simulink library "Susp_LUT"  (R2023b)
settings: Solver=VariableStepAuto  StartTime=0.0  StopTime=10.0  RelTol=1e-3
undefined symbols (not defined in the file or in its folder): Axle1D, AxleIn, Init, RaceFix, RaceSpin, Susp, Visual, X, Y, Z
libraries: Susp_DOF15 x5, LUT_Susp_Lib x2, sm_lib x2, Suspension_Utilities x2, Steer_Ackermann x1, Steer_Control_Axle2 x1
Description:
  | Component of Simscape Vehicle Templates Library
  | 
  | Copyright 2018-2026 The MathWorks, Inc.
settings Model: Creator=smiller  LastModifiedBy=smiller
settings ModelReferenceCC: EnableRefExpFcnMdlSchedulingChecks=on

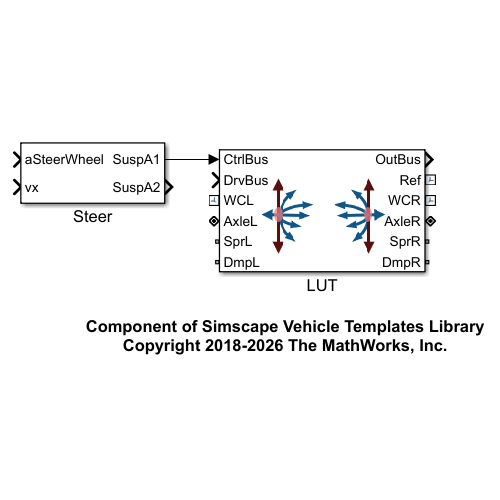
[thumbnail: Simulink's stored preview of the top-level diagram]
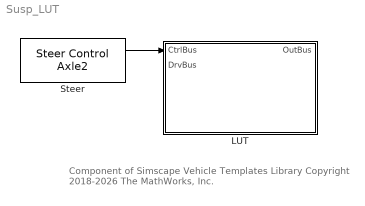
== system Susp_LUT ==
  note: Component of Simscape Vehicle Templates Library
      | Copyright 2018-2026 The MathWorks, Inc.
  LUT : Subsystem  mask(LUT Suspension with Optional Compliance and Steering){}
      mask help: Models suspension kinematics defined using a lookup table. The wheel frame lateral position, longitudinal position, and orientation are defined based on the height of the wheel frame. An optional 6-DOF compliance is placed at the wheel frame. Steering can be enabled.
      mask Display: image('sm_car_vehicle_susp_lut_IMAGE.png');
  Steer : Steer_Control_Axle2/Steer Control Axle2  Steer=Control.Default.Steer
  wires:
  Steer/1 -> LUT/1(CtrlBus)

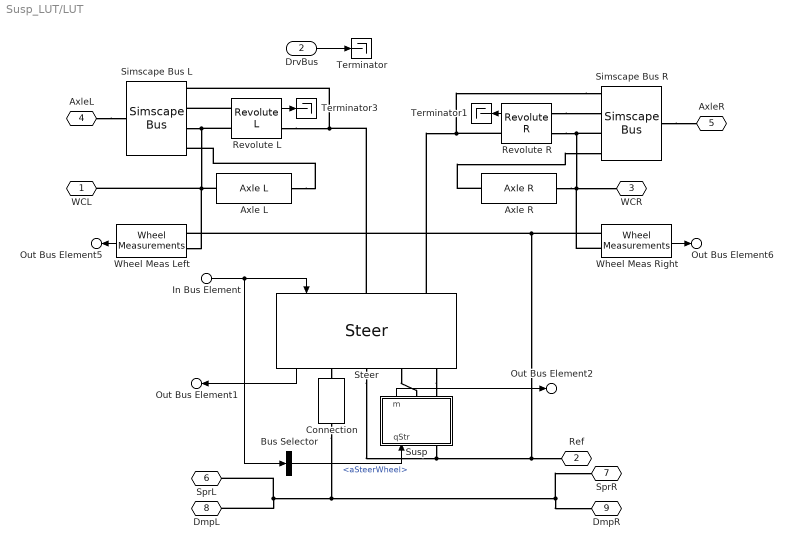
== system Susp_LUT/LUT ==
  In Bus Element : Inport  PortName=CtrlBus  Element=Steer
  DrvBus : Inport  Port=2
  Axle L : Susp_DOF15/Simple/Axle L  axle_len=Susp.LUT.Axle.xAxle.Value  axle_mass=Susp.LUT.Axle.mAxle.Value  clr_axle=Visual.Axle.clr  opc_axle=Visual.part.opc  radius_axle=Visual.Axle.rad
  Axle R : Susp_DOF15/Simple/Axle R  axle_len=Susp.LUT.Axle.xAxle.Value  axle_mass=Susp.LUT.Axle.mAxle.Value  clr_axle=Visual.Axle.clr  opc_axle=Visual.part.opc  radius_axle=Visual.Axle.rad
  Bus Selector : BusSelector  OutputSignals=aSteerWheel
  Connection : Susp_DOF15/Simple/Connection  SystemSampleTime=-1  VariantActivationTime=update diagram  AllowFlexibleInterface=on  Latency=0  AutoFrameSizeCalculation=off
  Revolute L : Susp_DOF15/Simple/Revolute L  whl_spd_init_jnt=Init.nWheel.Value(1)
  Revolute R : Susp_DOF15/Simple/Revolute R  whl_spd_init_jnt=Init.nWheel.Value(2)
  Simscape Bus L : SimscapeBus  HierarchyStrings=RaceFix;Axle1D;RaceSpin;AxleIn
  Simscape Bus R : SimscapeBus  HierarchyStrings=RaceFix;Axle1D;RaceSpin;AxleIn
  Steer : Steer_Ackermann/Steer  VariantControl=Variant1  LabelModeActiveChoice=Ackermann  Steer=Susp.Steer  VariantLabel=Susp.Steer.class.Value
      settings: AttributesFormatString=%<ActiveVariant>
  Susp : Subsystem  mask{kin_qz_vec=Susp.LUT.Kinematics.aToe.Value, kin_zvec_qz=Susp.LUT.Kinematics.zaToe.Value, kin_qy_vec=Susp.LUT.Kinematics.aCaster.Value, kin_zvec_qy=Susp.LUT.Kinematics.zaCaster.Value, kin_qx_vec=Susp.LUT.Kinematics.aCamber.Value, kin_zvec_qx=Susp.LUT.Kinematics.zaCamber.Value, kin_px_vec=Susp.LUT.Kinematics.xLong.Value, kin_zvec_px=Susp.LUT.Kinematics.zxLong.Value, kin_py_vec=Susp.LUT.Kinematics.xLat.Value, kin_zvec_py=Susp.LUT.Kinematics.zxLat.Value, kin_fz_vec=Susp.LUT.Spring.f.Value, kin_zvec_fz=Susp.LUT.Spring.x.Value, kin_vr_vec=Susp.LUT.Spring.vrt.Value, kin_zvec_vr=Susp.LUT.Spring.zvrt.Value, spring_b=Susp.LUT.Spring.d.Value, kin_tFilt=Susp.LUT.Kinematics.tFiltKin.Value, tFilt_pz=Susp.LUT.Kinematics.tFiltPz.Value, Compliance=Susp.LUT.Compliance, hp_wheel_ctr=Susp.LUT.Wheel.sWheelCentre.Value, mUnsprungMass=Susp.LUT.UnsprungMass.m.Value, JUnsprungMass=Susp.LUT.UnsprungMass.J.Value, aCaster=Susp.LUT.Steer.aCaster.Value, aKPI=Susp.LUT.Steer.aKPI.Value}
      mask prompts: spring_b "Damping (N/m/s))"; kin_tFilt "Filter Time Constant Kinematics (s)"; tFilt_pz "Filter Time Constant, Height (s)"; hp_wheel_ctr "HP Wheel Center [x y z] (m)"; mUnsprungMass "Unsprung Mass (kg)"; JUnsprungMass "Unsprung Inertia (kg*m^2)"; aCaster "Caster Angle (deg)"; aKPI "King Pin Inclination (KPI) Angle (deg)"
      mask TypeOptions kin_qz_vec: SuspL/kin_qz_vec | SuspR/kin_qz_vec
      mask TypeOptions kin_zvec_qz: SuspL/kin_zvec_qz | SuspR/kin_zvec_qz
      mask TypeOptions kin_qy_vec: SuspL/kin_qy_vec | SuspR/kin_qy_vec
      mask TypeOptions kin_zvec_qy: SuspL/kin_zvec_qy | SuspR/kin_zvec_qy
      mask TypeOptions kin_qx_vec: SuspL/kin_qx_vec | SuspR/kin_qx_vec
      mask TypeOptions kin_zvec_qx: SuspL/kin_zvec_qx | SuspR/kin_zvec_qx
      mask TypeOptions kin_px_vec: SuspL/kin_px_vec | SuspR/kin_px_vec
      mask TypeOptions kin_zvec_px: SuspL/kin_zvec_px | SuspR/kin_zvec_px
      mask TypeOptions kin_py_vec: SuspL/kin_py_vec | SuspR/kin_py_vec
      mask TypeOptions kin_zvec_py: SuspL/kin_zvec_py | SuspR/kin_zvec_py
      mask TypeOptions kin_fz_vec: SuspL/kin_fz_vec | SuspR/kin_fz_vec
      mask TypeOptions kin_zvec_fz: SuspL/kin_zvec_fz | SuspR/kin_zvec_fz
      mask TypeOptions kin_vr_vec: SuspL/kin_vr_vec | SuspR/kin_vr_vec
      mask TypeOptions kin_zvec_vr: SuspL/kin_zvec_vr | SuspR/kin_zvec_vr
      mask TypeOptions spring_b: SuspL/spring_b | SuspR/spring_b
      mask TypeOptions kin_tFilt: SuspL/kin_tFilt | SuspR/kin_tFilt
      mask TypeOptions tFilt_pz: SuspL/tFilt_pz | SuspR/tFilt_pz
      mask TypeOptions Compliance: SuspL/Compliance | SuspR/Compliance
      mask TypeOptions mUnsprungMass: SuspL/mUnsprungMass | SuspR/mUnsprungMass
      mask TypeOptions JUnsprungMass: SuspL/JUnsprungMass | SuspR/JUnsprungMass
      mask TypeOptions aCaster: SuspL/aCaster | SuspR/aCaster
      mask TypeOptions aKPI: SuspL/aKPI | SuspR/aKPI
      mask DialogControl cont_kinematics Prompt: Kinematics
      mask DialogControl text_kin_value Prompt: Value
      mask DialogControl text_kin_height Prompt: Height (m)
      mask DialogControl text_kin_zvec_qz Prompt: Toe Angle (deg)
      mask DialogControl text_kin_qy_vec Prompt: Caster Angle (deg)
      mask DialogControl text_kin_qx_vec Prompt: Camber Angle (deg)
      mask DialogControl text_kin_px_vec Prompt: Longitud. Pos. (m)
      mask DialogControl text_kin_py_vec Prompt: Lateral Position (m)
      mask DialogControl text_kin_fz_vec Prompt: Spring Force (N)
      mask DialogControl text_kin_vr_vec Prompt: Velocity Ratio (1)
      mask DialogControl cont_cpl Prompt: Compliance
      mask DialogControl cont_dim Prompt: Dimensions
      mask DialogControl cont_steer Prompt: Steer
  Terminator : Terminator
  Terminator1 : Terminator
  Terminator3 : Terminator
  Wheel Meas Left : Suspension_Utilities/Wheel Measurements  popup_leftRight=Left
  Wheel Meas Right : Suspension_Utilities/Wheel Measurements  popup_leftRight=Right
  WCL : PMIOPort  Side=Left
  Ref : PMIOPort  Port=2  Side=Right
  WCR : PMIOPort  Port=3  Side=Right
  AxleL : PMIOPort  Port=4  Side=Left
  AxleR : PMIOPort  Port=5  Side=Right
  SprL : PMIOPort  Port=6  Side=Left
  SprR : PMIOPort  Port=7  Side=Right
  DmpL : PMIOPort  Port=8  Side=Left
  DmpR : PMIOPort  Port=9  Side=Right
  Out Bus Element1 : Outport  VectorParamsAs1DForOutWhenUnconnected=off  PortName=OutBus  Element=Steer
  Out Bus Element5 : Outport  VectorParamsAs1DForOutWhenUnconnected=off  PortName=OutBus  Element=WhlL
  Out Bus Element6 : Outport  VectorParamsAs1DForOutWhenUnconnected=off  PortName=OutBus  Element=WhlR
  Out Bus Element2 : Outport  VectorParamsAs1DForOutWhenUnconnected=off  PortName=OutBus  Element=LUT
  wires:
  Wheel Meas Left/1 -> Out Bus Element5/1
  In Bus Element/1 -> Steer/1, Bus Selector/1
  Revolute L/1 -> Terminator3/1
  Bus Selector/1 -> Susp/1(qStr)  "<aSteerWheel>"
  Revolute R/1 -> Terminator1/1
  DrvBus/1 -> Terminator/1
  Steer/1 -> Out Bus Element1/1
  Wheel Meas Right/1 -> Out Bus Element6/1
  Susp/1(m) -> Out Bus Element2/1
  connections:
  DmpL/RConn1 -- SprL/RConn1 -- Connection/RConn1 -- DmpR/RConn1 -- SprR/RConn1
  Revolute R/LConn1 -- Simscape Bus R/LConn2
  Axle R/LConn1 -- WCR/RConn1 -- Wheel Meas Right/LConn2 -- Revolute R/LConn2 -- Simscape Bus R/LConn3
  Axle L/LConn1 -- WCL/RConn1 -- Simscape Bus L/LConn3 -- Revolute L/LConn2 -- Wheel Meas Left/LConn2
  Wheel Meas Right/LConn1 -- Wheel Meas Left/LConn1 -- Steer/RConn2 -- Susp/LConn1 -- Ref/RConn1
  Simscape Bus L/LConn1 -- Steer/LConn1 -- Revolute L/RConn1
  Steer/RConn3 -- Susp/RConn1
  Steer/RConn4 -- Susp/RConn2
  Steer/RConn1 -- Connection/LConn1
  Revolute L/LConn1 -- Simscape Bus L/LConn2
  Simscape Bus R/LConn1 -- Steer/LConn2 -- Revolute R/RConn1
  AxleL/RConn1 -- Simscape Bus L/RConn1
  Simscape Bus R/RConn1 -- AxleR/RConn1
  Axle L/RConn1 -- Simscape Bus L/LConn4
  Axle R/RConn1 -- Simscape Bus R/LConn4

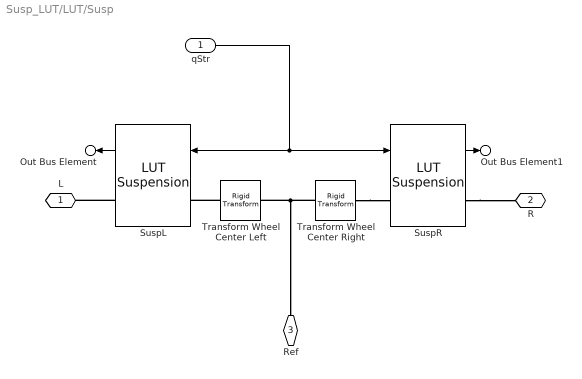
== system Susp_LUT/LUT/Susp ==
  qStr : Inport
  SuspL : LUT_Susp_Lib/LUT Suspension  popup_leftRight=Left  kin_qz_vec=kin_qz_vec  kin_zvec_qz=kin_zvec_qz  kin_qy_vec=kin_qy_vec  kin_zvec_qy=kin_zvec_qy  kin_qx_vec=kin_qx_vec  kin_zvec_qx=kin_zvec_qx  kin_px_vec=kin_px_vec  kin_zvec_px=kin_zvec_px  kin_py_vec=kin_py_vec  kin_zvec_py=kin_zvec_py  kin_fz_vec=kin_fz_vec  kin_zvec_fz=kin_zvec_fz  kin_vr_vec=kin_vr_vec  kin_zvec_vr=kin_zvec_vr  spring_b=spring_b  kin_tFilt=kin_tFilt  tFilt_pz=tFilt_pz  Compliance=Compliance  checkbox_setTargets=on  shell_or=Visual.hp.rad*2  elastomer_ir=Visual.hp.rad  shell_len=Visual.hp.rad*2  elastomer_clr=Visual.Bushing.clr  elastomer_opc=Visual.part.opc  elastomer_axis_clr=Visual.BushingXAxis.clr  mUnsprungMass=mUnsprungMass  JUnsprungMass=JUnsprungMass  aCaster=aCaster  aKPI=aKPI
  SuspR : LUT_Susp_Lib/LUT Suspension  popup_leftRight=Right  kin_qz_vec=kin_qz_vec  kin_zvec_qz=kin_zvec_qz  kin_qy_vec=kin_qy_vec  kin_zvec_qy=kin_zvec_qy  kin_qx_vec=kin_qx_vec  kin_zvec_qx=kin_zvec_qx  kin_px_vec=kin_px_vec  kin_zvec_px=kin_zvec_px  kin_py_vec=kin_py_vec  kin_zvec_py=kin_zvec_py  kin_fz_vec=kin_fz_vec  kin_zvec_fz=kin_zvec_fz  kin_vr_vec=kin_vr_vec  kin_zvec_vr=kin_zvec_vr  spring_b=spring_b  kin_tFilt=kin_tFilt  tFilt_pz=tFilt_pz  Compliance=Compliance  checkbox_setTargets=on  shell_or=Visual.hp.rad*2  elastomer_ir=Visual.hp.rad  shell_len=Visual.hp.rad*2  elastomer_clr=Visual.Bushing.clr  elastomer_opc=Visual.part.opc  elastomer_axis_clr=Visual.BushingXAxis.clr  mUnsprungMass=mUnsprungMass  JUnsprungMass=JUnsprungMass  aCaster=aCaster  aKPI=aKPI
  Transform Wheel Center Left : sm_lib/Frames and Transforms/Rigid Transform  TranslationMethod=Cartesian  TranslationStandardOffset=0  TranslationStandardOffsetUnits=m  TranslationStandardAxis=+Z  TranslationCartesianOffset=hp_wheel_ctr  TranslationCartesianOffsetUnits=m  TranslationROffset=0  TranslationROffsetUnits=m  TranslationZOffset=0  TranslationZOffsetUnits=m  TranslationThetaOffset=0  TranslationThetaOffsetUnits=deg  RotationMethod=None  RotationAngleUnits=deg  RotationStandardAxis=+Z  RotationAngle=0.0  RotationArbitraryAxis=[0 0 1]  FollAlignAxisA=+X  BaseAlignAxisA=+Y  FollAlignAxisB=+Y  BaseAlignAxisB=+Z  RotationSequenceAxes=FollowerAxes  RotationSequence=XYX  RotationSequenceAngles=[0 0 0]  RotationSequenceAnglesUnits=deg  RotationMatrix=[1 0 0; 0 1 0; 0 0 1]  Quaternion=[1 0 0 0]
  Transform Wheel Center Right : sm_lib/Frames and Transforms/Rigid Transform  TranslationMethod=Cartesian  TranslationStandardOffset=0  TranslationStandardOffsetUnits=m  TranslationStandardAxis=+Z  TranslationCartesianOffset=hp_wheel_ctr.*[1 -1 1]  TranslationCartesianOffsetUnits=m  TranslationROffset=0  TranslationROffsetUnits=m  TranslationZOffset=0  TranslationZOffsetUnits=m  TranslationThetaOffset=0  TranslationThetaOffsetUnits=deg  RotationMethod=None  RotationAngleUnits=deg  RotationStandardAxis=+Z  RotationAngle=0.0  RotationArbitraryAxis=[0 0 1]  FollAlignAxisA=+X  BaseAlignAxisA=+Y  FollAlignAxisB=+Y  BaseAlignAxisB=+Z  RotationSequenceAxes=FollowerAxes  RotationSequence=XYX  RotationSequenceAngles=[0 0 0]  RotationSequenceAnglesUnits=deg  RotationMatrix=[1 0 0; 0 1 0; 0 0 1]  Quaternion=[1 0 0 0]
  L : PMIOPort  Side=Right
  R : PMIOPort  Port=2  Side=Right
  Ref : PMIOPort  Port=3  Side=Left
  Out Bus Element : Outport  PortName=m  Element=SuspL
  Out Bus Element1 : Outport  PortName=m  Element=SuspR
  wires:
  qStr/1 -> SuspR/1, SuspL/1
  SuspL/1 -> Out Bus Element/1
  SuspR/1 -> Out Bus Element1/1
  connections:
  SuspL/RConn1 -- L/RConn1
  Transform Wheel Center Right/LConn1 -- Ref/RConn1 -- Transform Wheel Center Left/LConn1
  SuspR/RConn1 -- R/RConn1
  Transform Wheel Center Left/RConn1 -- SuspL/LConn1
  Transform Wheel Center Right/RConn1 -- SuspR/LConn1
